simulink model "discreteInner"  (R2020b)
settings: Solver=VariableStepAuto  StartTime=0.0  StopTime=inf  RelTol=2.8421709430404007E-14
values from neighbouring files (symbols this model uses):
  dt_delay = 0.011    [main.m]
  dt_sample = 0.01    [main.m]
  Kd = diag([K1d; K2d; K3d])    [main.m]
  wbi0_B = [0;0;0]    [main.m]
  wbistar_B = timeseries(stepf,0:0.01:20)    [main.m]
undefined symbols (not defined in the file or in its folder): A_BP, A_PB, J_C_B, q0_BI
libraries: dspnetwork x4
settings Model: EnablePacing=on  Creator=bbingham  LastModifiedBy=tjones
settings DataIOCC: SaveOutput=off  SignalLogging=off  DSMLogging=off  ReturnWorkspaceOutputs=off
settings DebuggingCC: ArithmeticOperatorsInVariantConditions=warning
settings SFSimCC: SimUseLocalCustomCode=off  CustomCodeUndefinedFunction=UseInterfaceOnly
settings RTWCC: Description=Simulink Desktop Real-Time  SystemTargetFile=sldrt.tlc  TemplateMakefile=sldrt.tmf  RTWUseLocalCustomCode=off  RTWCompilerOptimization=on
settings CodeAppCC: MaxIdLength=95  StateflowObjectComments=on
settings TargetCC: TargetPreCompLibLocation=C:\Program Files\MATLAB\R2020a\toolbox\sldrt\lib\win64  TargetLangStandard=C99 (ISO)  SupportVariableSizeSignals=on
settings SimscapeCC: SimscapeNormalizeSystem=off

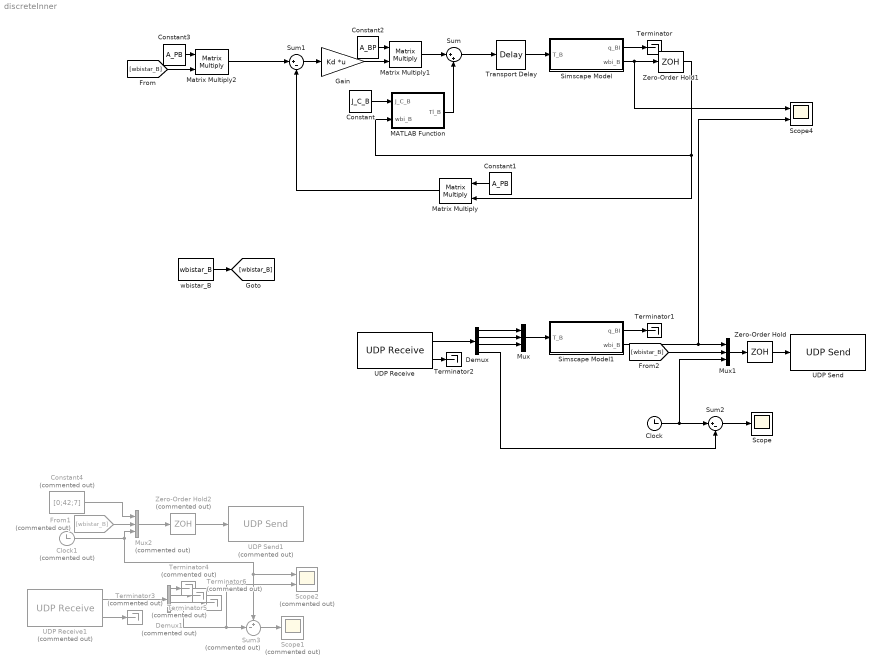
== system discreteInner ==
  Clock : Clock
  Clock1 : Clock  Commented=on
  Constant : Constant  Value=J_C_B  SampleTime=dt_sample
  Constant1 : Constant  Value=A_PB  SampleTime=dt_sample
  Constant2 : Constant  Value=A_BP  SampleTime=dt_sample
  Constant3 : Constant  Value=A_PB  SampleTime=dt_sample
  Constant4 : Constant  Commented=on  Value=[0;42;7]
  Demux : Demux
  Demux1 : Demux  Commented=on
  From1 : From  Commented=on  GotoTag=wbistar_B
  Gain : Gain  Gain=Kd  Multiplication=Matrix(K*u) (u vector)
  MATLAB Function : MATLAB Function  TreatAsAtomicUnit=on
  Matrix Multiply : Product  Multiplication=Matrix(*)
  Matrix Multiply1 : Product  Multiplication=Matrix(*)
  Matrix Multiply2 : Product  Multiplication=Matrix(*)
  Mux : Mux  Inputs=3
  Mux1 : Mux  Inputs=3
  Mux2 : Mux  Commented=on  Inputs=3
  Scope : Scope
  Scope1 : Scope  Commented=on
  Scope2 : Scope  Commented=on  NumInputPorts=2
  Scope4 : Scope  NumInputPorts=2
  Simscape Model : Subsystem  TreatAsAtomicUnit=on
  Simscape Model1 : Subsystem  TreatAsAtomicUnit=on
  Sum : Sum  Inputs=|++
  Sum1 : Sum  Inputs=|+-
  Sum2 : Sum  Inputs=|+-
  Sum3 : Sum  Commented=on  Inputs=+-|
  Terminator : Terminator
  Terminator1 : Terminator
  Terminator2 : Terminator
  Terminator{3..6} (4 alike) : Terminator  Commented=on
  Transport Delay : TransportDelay  DelayTime=dt_delay  BufferSize=2048
  UDP Receive : dspnetwork/UDP Receive  localURL='0.0.0.0'  localPort=12346  remoteURL='0.0.0.0'  remotePort=-1  recvBufferSize=8192  dims=4  signalDatatype=double  isComplex=off  isVarSize=off  showBlockingTime=off  blockingTime=0  sampletime=.001  blockPlatform=[]
  UDP Receive1 : dspnetwork/UDP Receive  Commented=on  localURL='0.0.0.0'  localPort=12346  remoteURL='0.0.0.0'  remotePort=-1  recvBufferSize=8192  dims=4  signalDatatype=double  isComplex=off  isVarSize=off  showBlockingTime=off  blockingTime=0  sampletime=.001  blockPlatform=[]
  UDP Send : dspnetwork/UDP Send  remoteURL='172.31.220.90'  remotePort=12345  localURL='0.0.0.0'  localPortSource=Automatically determine  localPort=-1  sendBufferSize=8192  sampletime=-1  blockPlatform=[]  separateLengthPort=0
  UDP Send1 : dspnetwork/UDP Send  Commented=on  remoteURL='172.31.220.90'  remotePort=12345  localURL='0.0.0.0'  localPortSource=Automatically determine  localPort=-1  sendBufferSize=8192  sampletime=-1  blockPlatform=[]  separateLengthPort=0
  Zero-Order Hold : ZeroOrderHold  SampleTime=dt_sample
  Zero-Order Hold1 : ZeroOrderHold  SampleTime=dt_sample
  Zero-Order Hold2 : ZeroOrderHold  Commented=on  SampleTime=dt_sample
  wbistar_B : Constant  Value=wbistar_B  SampleTime=dt_sample
  wires:
  Transport Delay/1 -> Simscape Model/1(T_B)
  Simscape Model/1(q_BI) -> Terminator/1
  Sum/1 -> Transport Delay/1
  Zero-Order Hold1/1 -> MATLAB Function/2(wbi_B), Matrix Multiply/2
  MATLAB Function/1(Tl_B) -> Sum/2
  Constant/1 -> MATLAB Function/1(J_C_B)
  Constant1/1 -> Matrix Multiply/1
  Matrix Multiply/1 -> Sum1/2
  Sum1/1 -> Gain/1
  Constant2/1 -> Matrix Multiply1/1
  Gain/1 -> Matrix Multiply1/2
  Matrix Multiply1/1 -> Sum/1
  Constant3/1 -> Matrix Multiply2/1
  Matrix Multiply2/1 -> Sum1/1
  Simscape Model/2(wbi_B) -> Scope4/1, Zero-Order Hold1/1
  Simscape Model1/1(q_BI) -> Terminator1/1
  UDP Receive/1 -> Demux/1
  Demux/1 -> Mux/1
  Demux/2 -> Mux/2
  Demux/3 -> Mux/3
  Mux/1 -> Simscape Model1/1(T_B)
  UDP Receive/2 -> Terminator2/1
  Simscape Model1/2(wbi_B) -> Scope4/2, Mux1/1
  [wbistar_B] -> Mux1/2
  Clock/1 -> Sum2/1, Mux1/3
  Demux/4 -> Sum2/2
  Sum2/1 -> Scope/1
  Mux1/1 -> Zero-Order Hold/1
  Zero-Order Hold/1 -> UDP Send/1
  UDP Receive1/2 -> Terminator3/1
  Zero-Order Hold2/1 -> UDP Send1/1
  Mux2/1 -> Zero-Order Hold2/1
  wbistar_B/1 -> [wbistar_B]
  [wbistar_B] -> Matrix Multiply2/2
  From1/1 -> Mux2/2
  Constant4/1 -> Mux2/1
  UDP Receive1/1 -> Demux1/1
  Demux1/4 -> Scope2/2, Sum3/2
  Sum3/1 -> Scope1/1
  Demux1/1 -> Terminator4/1
  Demux1/2 -> Terminator5/1
  Demux1/3 -> Terminator6/1
  Clock1/1 -> Scope2/1, Sum3/1, Mux2/3

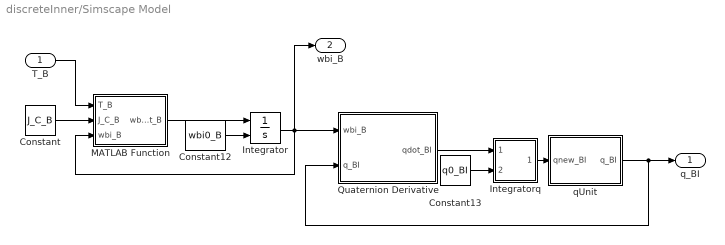
== system discreteInner/Simscape Model ==
  T_B : Inport
  Constant : Constant  Value=J_C_B
  Constant12 : Constant  Value=wbi0_B
  Constant13 : Constant  Value=q0_BI  OutDataTypeStr=Bus: qBus
  Integrator : Integrator  InitialConditionSource=external
  Integratorq : Subsystem
  MATLAB Function : MATLAB Function  TreatAsAtomicUnit=on
  Quaternion Derivative : MATLAB Function  TreatAsAtomicUnit=on
  qUnit : MATLAB Function  TreatAsAtomicUnit=on
  q_BI : Outport  OutDataTypeStr=Bus: qBus  VectorParamsAs1DForOutWhenUnconnected=off
  wbi_B : Outport  Port=2  VectorParamsAs1DForOutWhenUnconnected=off
  wires:
  qUnit/1(q_BI) -> q_BI/1, Quaternion Derivative/2(q_BI)
  Integratorq/1(qnew_BI) -> qUnit/1(qnew_BI)
  Quaternion Derivative/1(qdot_BI) -> Integratorq/1(qdot_BI)
  Constant13/1 -> Integratorq/2(q0_BI)
  MATLAB Function/1(wbidot_B) -> Integrator/1
  Constant12/1 -> Integrator/2
  Constant/1 -> MATLAB Function/2(J_C_B)
  Integrator/1 -> wbi_B/1, MATLAB Function/3(wbi_B), Quaternion Derivative/1(wbi_B)
  T_B/1 -> MATLAB Function/1(T_B)

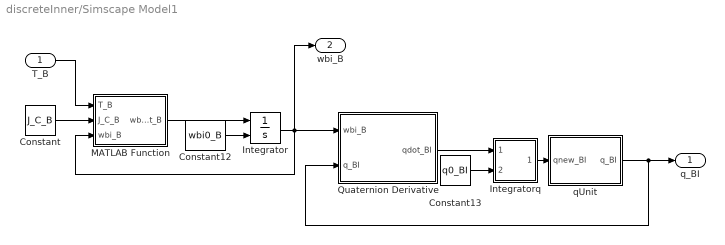
== system discreteInner/Simscape Model1 ==
  T_B : Inport
  Constant : Constant  Value=J_C_B
  Constant12 : Constant  Value=wbi0_B
  Constant13 : Constant  Value=q0_BI  OutDataTypeStr=Bus: qBus
  Integrator : Integrator  InitialConditionSource=external
  Integratorq : Subsystem
  MATLAB Function : MATLAB Function  TreatAsAtomicUnit=on
  Quaternion Derivative : MATLAB Function  TreatAsAtomicUnit=on
  qUnit : MATLAB Function  TreatAsAtomicUnit=on
  q_BI : Outport  OutDataTypeStr=Bus: qBus  VectorParamsAs1DForOutWhenUnconnected=off
  wbi_B : Outport  Port=2  VectorParamsAs1DForOutWhenUnconnected=off
  wires:
  T_B/1 -> MATLAB Function/1(T_B)
  Integrator/1 -> Quaternion Derivative/1(wbi_B), MATLAB Function/3(wbi_B), wbi_B/1
  Constant/1 -> MATLAB Function/2(J_C_B)
  Constant12/1 -> Integrator/2
  MATLAB Function/1(wbidot_B) -> Integrator/1
  Constant13/1 -> Integratorq/2(q0_BI)
  Quaternion Derivative/1(qdot_BI) -> Integratorq/1(qdot_BI)
  Integratorq/1(qnew_BI) -> qUnit/1(qnew_BI)
  qUnit/1(q_BI) -> Quaternion Derivative/2(q_BI), q_BI/1

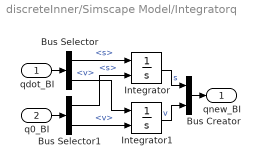
== system discreteInner/Simscape Model/Integratorq ==
  qdot_BI : Inport  OutDataTypeStr=Bus: qBus
  q0_BI : Inport  Port=2  OutDataTypeStr=Bus: qBus
  Bus Creator : BusCreator  Inputs=2  OutDataTypeStr=Bus: qBus
      settings: InheritFromInputs=off
  Bus Selector : BusSelector  OutputSignals=s,v
  Bus Selector1 : BusSelector  OutputSignals=s,v
  Integrator : Integrator  InitialConditionSource=external
  Integrator1 : Integrator  InitialConditionSource=external
  qnew_BI : Outport  OutDataTypeStr=Bus: qBus  VectorParamsAs1DForOutWhenUnconnected=off
  wires:
  qdot_BI/1 -> Bus Selector/1
  q0_BI/1 -> Bus Selector1/1
  Bus Selector/1 -> Integrator/1  "<s>"
  Bus Selector1/1 -> Integrator/2  "<s>"
  Bus Selector/2 -> Integrator1/1  "<v>"
  Bus Selector1/2 -> Integrator1/2  "<v>"
  Integrator/1 -> Bus Creator/1  "s"
  Integrator1/1 -> Bus Creator/2  "v"
  Bus Creator/1 -> qnew_BI/1

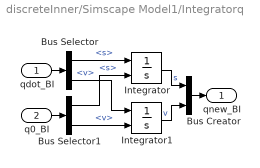
== system discreteInner/Simscape Model1/Integratorq ==
  qdot_BI : Inport  OutDataTypeStr=Bus: qBus
  q0_BI : Inport  Port=2  OutDataTypeStr=Bus: qBus
  Bus Creator : BusCreator  Inputs=2  OutDataTypeStr=Bus: qBus
      settings: InheritFromInputs=off
  Bus Selector : BusSelector  OutputSignals=s,v
  Bus Selector1 : BusSelector  OutputSignals=s,v
  Integrator : Integrator  InitialConditionSource=external
  Integrator1 : Integrator  InitialConditionSource=external
  qnew_BI : Outport  OutDataTypeStr=Bus: qBus  VectorParamsAs1DForOutWhenUnconnected=off
  wires:
  Bus Creator/1 -> qnew_BI/1
  Integrator1/1 -> Bus Creator/2  "v"
  Integrator/1 -> Bus Creator/1  "s"
  Bus Selector1/2 -> Integrator1/2  "<v>"
  Bus Selector/2 -> Integrator1/1  "<v>"
  Bus Selector1/1 -> Integrator/2  "<s>"
  Bus Selector/1 -> Integrator/1  "<s>"
  q0_BI/1 -> Bus Selector1/1
  qdot_BI/1 -> Bus Selector/1

== matlab function discreteInner/MATLAB Function ==
  data: J_C_B input; Tl_B output; wbi_B input
function Tl_B = fcn(J_C_B, wbi_B)

Tl_B = cross(wbi_B, J_C_B*wbi_B);

== matlab function discreteInner/Simscape Model/Quaternion Derivative ==
  data: wbi_B input; q_BI input Bus: qBus; qdot_BI output Bus: qBus
function qdot_BI = fcn(wbi_B, q_BI)

w.s = 0;
w.v = wbi_B;

qdot = qX(w, q_BI);

qdot_BI.s = 1/2*qdot.s;
qdot_BI.v = 1/2*qdot.v;

== matlab function discreteInner/Simscape Model1/MATLAB Function ==
  data: T_B input; wbidot_B output; J_C_B input; wbi_B input
function wbidot_B = fcn(T_B, J_C_B, wbi_B)

wbidot_B = J_C_B\(T_B - cross(wbi_B, J_C_B*wbi_B));

== matlab function discreteInner/Simscape Model1/Quaternion Derivative ==
  data: wbi_B input; q_BI input Bus: qBus; qdot_BI output Bus: qBus
function qdot_BI = fcn(wbi_B, q_BI)

w.s = 0;
w.v = wbi_B;

qdot = qX(w, q_BI);

qdot_BI.s = 1/2*qdot.s;
qdot_BI.v = 1/2*qdot.v;

== matlab function discreteInner/Simscape Model1/qUnit ==
  data: qnew_BI input Bus: qBus; q_BI output Bus: qBus
function q_BI = fcn(qnew_BI)

q_BI = qUnit(qnew_BI);

== matlab function discreteInner/Simscape Model/qUnit ==
  data: qnew_BI input Bus: qBus; q_BI output Bus: qBus
function q_BI = fcn(qnew_BI)

q_BI = qUnit(qnew_BI);

== matlab function discreteInner/Simscape Model/MATLAB Function ==
  data: T_B input; wbidot_B output; J_C_B input; wbi_B input
function wbidot_B = fcn(T_B, J_C_B, wbi_B)

wbidot_B = J_C_B\(T_B - cross(wbi_B, J_C_B*wbi_B));
